simulink model "Low_Pass_Filter"  (R2017a)
settings: Solver=FixedStepAuto  StartTime=0.0  StopTime=10.0  FixedStep=0.01  RelTol=1e-3
settings Model: Creator=LocalAccount  LastModifiedBy=LocalAccount

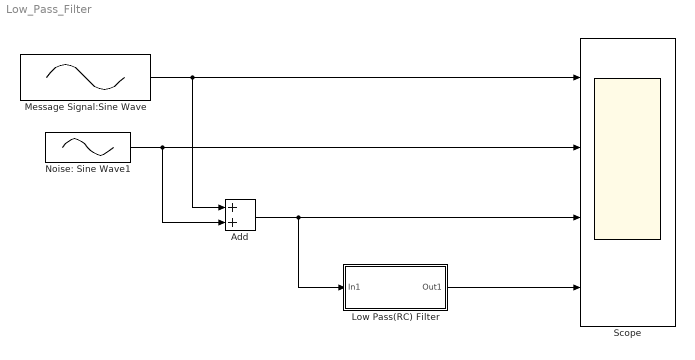
== system Low_Pass_Filter ==
  Add : Sum
  Low Pass(RC) Filter : Subsystem
  Message Signal:Sine Wave : Sin  Amplitude=100  Frequency=10  SampleTime=0
  Noise: Sine Wave1 : Sin  Amplitude=5  Frequency=100  SampleTime=0
  Scope : Scope  NumInputPorts=4
  wires:
  Low Pass(RC) Filter/1(Out1) -> Scope/4
  Add/1 -> Low Pass(RC) Filter/1(In1), Scope/3
  Message Signal:Sine Wave/1 -> Add/1, Scope/1
  Noise: Sine Wave1/1 -> Add/2, Scope/2

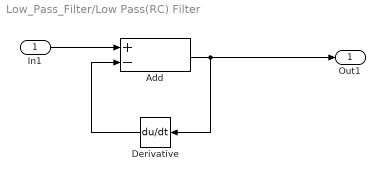
== system Low_Pass_Filter/Low Pass(RC) Filter ==
  In1 : Inport
  Add : Sum  Inputs=+-
  Derivative : Derivative
  Out1 : Outport
  wires:
  In1/1 -> Add/1
  Add/1 -> Derivative/1, Out1/1
  Derivative/1 -> Add/2
